simulink model "slexFMCWExample"  (R2018b)
settings: Solver=FixedStepDiscrete  StartTime=0.0  StopTime=20*64*paramFMCW.T  RelTol=1e-3  EnableMultiTasking=on
PreLoadFcn:
  | helperslexFMCWParam
undefined symbols (not defined in the file or in its folder): paramFMCW, physconst
libraries: phasedenvlib x6, phasedtxrxlib x2, phaseddetectlib x2, phasedwavlib x1, phasedmisclib x1
CloseFcn:
  | clear paramFMCW
Description:
  | FMCW Radar Range Estimation
  | 
  | This model shows how to use a FMCW radar to estimate a target's range.
settings Model: Creator=The MathWorks, Inc.  LastModifiedBy=The MathWorks, Inc.
settings DataIOCC: LimitDataPoints=on  SaveFormat=Array
settings OptimizationCC: LifeSpan=inf
settings DebuggingCC: ReadBeforeWriteMsg=DisableAll  WriteAfterWriteMsg=DisableAll  WriteAfterReadMsg=DisableAll  UnderspecifiedInitializationDetection=Classic  MergeDetectMultiDrivingBlocksExec=none  SolverPrmCheckMsg=warning  MultiTaskDSMMsg=none  AllowSymbolicDim=off  SFUnexpectedBacktrackingDiag=warning  SFNoUnconditionalDefaultTransitionDiag=warning  SFExecutionAtInitializationDiag=none
settings HardwareCC: ProdBitPerPointer=32  ProdBitPerSizeT=32  ProdBitPerPtrDiffT=32  ProdLargestAtomicFloat=None  ProdIntDivRoundTo=Undefined  ProdEndianess=Unspecified  ProdWordSize=32  ProdHWDeviceType=32-bit Generic
settings ModelReferenceCC: UpdateModelReferenceTargets=IfOutOfDate  PropagateSignalLabelsOutOfModel=off
settings SFSimCC: SFSimEcho=off  SimUseLocalCustomCode=off
settings RTWCC: RTWUseLocalCustomCode=off
settings CodeAppCC: StateflowObjectComments=on
settings GRTTargetCC: TargetLangStandard=C89/C90 (ANSI)  GeneratePreprocessorConditionals=Disable all
settings ConfigComp: CovMetricSettings=dw  CovHtmlReporting=on  CovSaveCumulativeToWorkspaceVar=on  CovSaveSingleToWorkspaceVar=on  CovExternalEMLEnable=off  CovSFcnEnable=off

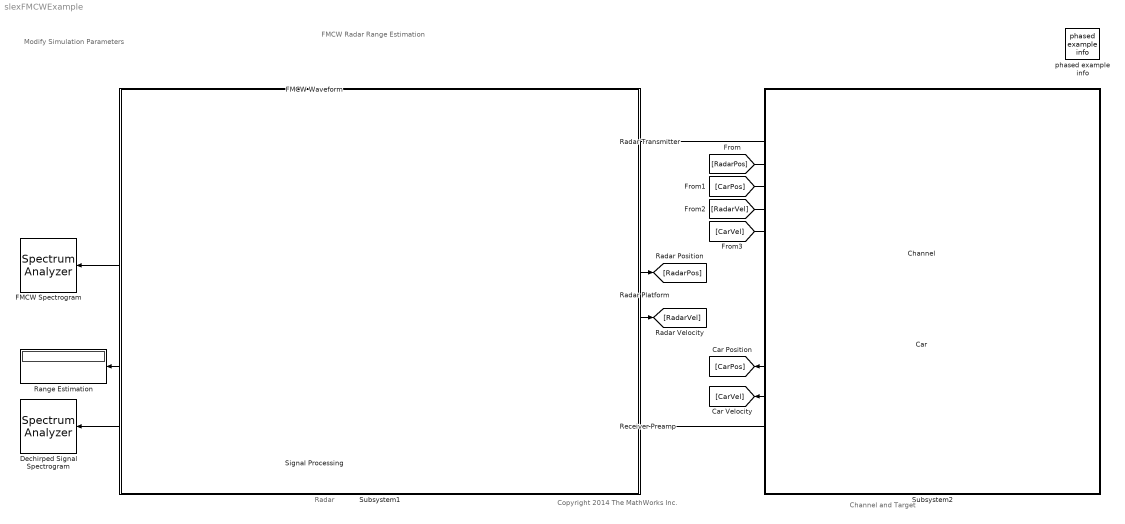
== system slexFMCWExample ==
  note: Copyright 2014 The MathWorks Inc.
  note: Radar
  note: Channel and Target
  note: FMCW Radar Range Estimation
  note: Modify Simulation Parameters
  Car : Subsystem
      mask Display:
      | disp('Car')
      | port_label('output',1,'Pos')
      | port_label('output',2,'Vel')
      | port_label('output',3,'Sig')
  Channel : Subsystem  VariantControlMode=Label  Variant=on  LabelModeActiveChoice=FreeSpace  mask{ChannelSelection=Free space}
      mask prompts: ChannelSelection "Propagation Channel"
      mask init:
      | cstr = get_param(gcb,'ChannelSelection');
      | if strcmp(cstr,'Free space')
      |     set_param(gcb,'OverrideUsingVariant','FreeSpace');
      | else
      |     set_param(gcb,'OverrideUsingVariant','TwoRay');
      | end
      mask TypeOptions ChannelSelection: Free space | Two-ray
      mask DialogControl DescGroupVar Prompt: Channel
      mask DialogControl DescTextVar Prompt: Propagation channel between the radar and the car
      mask Display:
      | port_label('output',1,'y')
      | port_label('input',1,'x')
      | port_label('input',2,'pos1')
      | port_label('input',3,'pos2')
      | port_label('input',4,'vel1')
      | port_label('input',5,'vel2')
      | disp('Channel')
  Dechirped Signal Spectrogram : SpectrumAnalyzer
  FMCW Spectrogram : SpectrumAnalyzer
  FMCW Waveform : phasedwavlib/FMCW Waveform  SampleRate=paramFMCW.Fs  SweepTime=paramFMCW.T  SweepBandwidth=paramFMCW.Fs  SweepDirection=Up  SweepInterval=Symmetric  OutputFormat=Sweeps  NumSamples=100  NumSweeps=1  SimulateUsing=Interpreted execution
      settings: SourceProductName=Phased Array System Toolbox  SourceProductBaseCode=AR
  Radar Platform : phasedenvlib/Motion Platform  MotionModel=Velocity  InitialPosition=paramFMCW.RadarPos  InitialVelocity=[ 0; 0; 0 ]  VelocitySource=Property  Velocity=paramFMCW.RadarVel  AccelerationSource=Property  Acceleration=[0;0;0]  CustomTrajectory=[ 0, 0, 0, 0, 0, 0, 0; 1, 0, 0, 0, 0, 0, 0 ]  ScanMode=None  InitialScanAngle=0  AzimuthSpan=[ -60, 60 ]  AzimuthScanRate=10  InitialOrientationAxes=eye( 3 )  OrientationAxesOutputPort=off  ElapsedTimeSource=Auto  SampleRateFromInputCheckbox=on  SampleRate=1e6  SimulateUsing=Interpreted execution
      settings: SourceProductName=Phased Array System Toolbox  SourceProductBaseCode=AR
  Radar Transmitter : phasedtxrxlib/Transmitter  PeakPower=paramFMCW.ppow  Gain=paramFMCW.TxGain  LossFactor=0  InUseOutputPort=off  CoherentOnTransmit=on  PhaseNoiseOutputPort=off  SeedSource=Auto  Seed=0  SimulateUsing=Interpreted execution
      settings: SourceProductName=Phased Array System Toolbox  SourceProductBaseCode=AR
  Range Estimation : Display
  Receiver Preamp : phasedtxrxlib/Receiver Preamp  Gain=paramFMCW.RxGain  LossFactor=0  NoiseMethod=Noise temperature  NoiseFigure=paramFMCW.NF  ReferenceTemperature=290  SampleRateFromInputCheckbox=on  SampleRate=1e6  NoisePower=0  EnableInputPort=off  PhaseNoiseInputPort=off  SeedSource=Auto  Seed=0  SimulateUsing=Interpreted execution
      settings: SourceProductName=Phased Array System Toolbox  SourceProductBaseCode=AR
  Signal Processing : Subsystem
      mask Display:
      | disp('Signal Processing')
      | port_label('input',1,'Ref')
      | port_label('input',2,'Echo')
      | port_label('output',1,'Rng')
      | port_label('output',2,'Dechirped')
  Subsystem1 : Subsystem
  Subsystem2 : Subsystem
  phased example info : phasedmisclib/phased example info  SystemSampleTime=-1
      settings: SourceProductName=Phased Array System Toolbox  SourceProductBaseCode=AR
  wires:
  FMCW Waveform/1 -> Signal Processing/1(In1), FMCW Spectrogram/1, Radar Transmitter/1
  Radar Platform/1 -> [RadarPos]
  Radar Platform/2 -> [RadarVel]
  Car/1(Out1) -> [CarPos]
  Car/2(Out2) -> [CarVel]
  Car/3(Out3) -> Receiver Preamp/1
  Receiver Preamp/1 -> Signal Processing/2(In2)
  Signal Processing/1(Out1) -> Range Estimation/1
  Signal Processing/2(Out2) -> Dechirped Signal Spectrogram/1
  Radar Transmitter/1 -> Channel/1(In1)
  [RadarPos] -> Channel/2(In2)
  [CarPos] -> Channel/3(In3)
  [RadarVel] -> Channel/4(In4)
  [CarVel] -> Channel/5(In5)
  Channel/1(Out1) -> Car/1(In1)

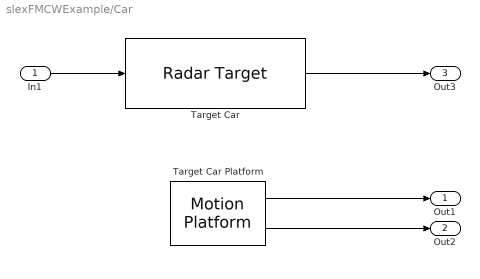
== system slexFMCWExample/Car ==
  In1 : Inport
  Target Car : phasedenvlib/Radar Target  EnablePolarization=off  Mode=Monostatic  MeanRCSSource=Property  ScatteringMatrixSource=Property  MeanRCS=paramFMCW.RCS  ScatteringMatrix=eye( 2 )  Model=Nonfluctuating  PropagationSpeed=paramFMCW.C  OperatingFrequency=paramFMCW.Fc  SeedSource=Auto  Seed=0  SimulateUsing=Interpreted execution
      settings: SourceProductName=Phased Array System Toolbox  SourceProductBaseCode=AR
  Target Car Platform : phasedenvlib/Motion Platform  MotionModel=Velocity  InitialPosition=paramFMCW.CarPos  InitialVelocity=[ 0; 0; 0 ]  VelocitySource=Property  Velocity=paramFMCW.CarVel  AccelerationSource=Property  Acceleration=[0;0;0]  CustomTrajectory=[ 0, 0, 0, 0, 0, 0, 0; 1, 0, 0, 0, 0, 0, 0 ]  ScanMode=None  InitialScanAngle=0  AzimuthSpan=[ -60, 60 ]  AzimuthScanRate=10  InitialOrientationAxes=eye( 3 )  OrientationAxesOutputPort=off  ElapsedTimeSource=Auto  SampleRateFromInputCheckbox=on  SampleRate=1e6  SimulateUsing=Interpreted execution
      settings: SourceProductName=Phased Array System Toolbox  SourceProductBaseCode=AR
  Out1 : Outport
  Out2 : Outport  Port=2
  Out3 : Outport  Port=3
  wires:
  Target Car/1 -> Out3/1
  In1/1 -> Target Car/1
  Target Car Platform/1 -> Out1/1
  Target Car Platform/2 -> Out2/1

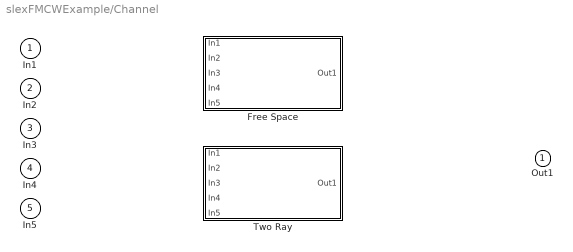
== system slexFMCWExample/Channel ==
  In1 : Inport
  In2 : Inport  Port=2
  In3 : Inport  Port=3
  In4 : Inport  Port=4
  In5 : Inport  Port=5
  Free Space : Subsystem  VariantControl=FreeSpace
      mask Display:
      | port_label('output',1,'y')
      | port_label('input',1,'x')
      | port_label('input',2,'pos1')
      | port_label('input',3,'pos2')
      | port_label('input',4,'vel1')
      | port_label('input',5,'vel2')
      | disp('Free Space')
  Two Ray : Subsystem  VariantControl=TwoRay
      mask Display:
      | port_label('output',1,'y')
      | port_label('input',1,'x')
      | port_label('input',2,'pos1')
      | port_label('input',3,'pos2')
      | port_label('input',4,'vel1')
      | port_label('input',5,'vel2')
      | disp('Two-Ray')
  Out1 : Outport

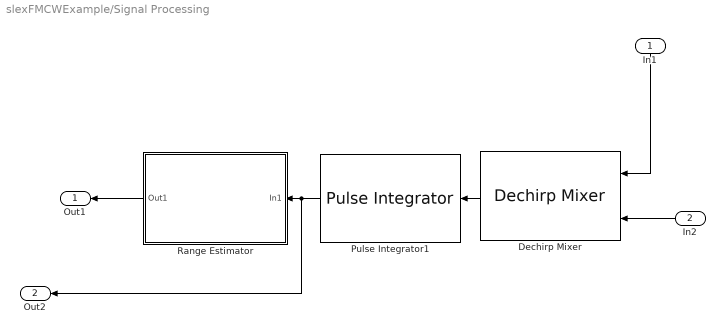
== system slexFMCWExample/Signal Processing ==
  In1 : Inport
  In2 : Inport  Port=2
  Dechirp Mixer : phaseddetectlib/Dechirp Mixer
      settings: SourceProductName=Phased Array System Toolbox  SourceProductBaseCode=AR
  Pulse Integrator1 : phaseddetectlib/Pulse Integrator  CoherentFlag=Coherent  N=64  V=0
      settings: SourceProductName=Phased Array System Toolbox  SourceProductBaseCode=AR
  Range Estimator : Subsystem  mask(Range Estimator){c=paramFMCW.C, k=paramFMCW.Fs/paramFMCW.T, N=2048}
      mask prompts: c "Propagation Speed (m/s)"; k "FMCW Sweep Slope (Hz/s)"; N "Number of FFT Points"
      mask help: Compute periodogram of the incoming signal, find the beat frequency, and convert the beat frequency to the range estimate.
      mask Display:
      | disp('Range\nEstimator')
      | port_label('input',1,'X')
      | port_label('output',1,'Rng')
  Out1 : Outport
  Out2 : Outport  Port=2
  wires:
  In1/1 -> Dechirp Mixer/1
  Dechirp Mixer/1 -> Pulse Integrator1/1
  In2/1 -> Dechirp Mixer/2
  Pulse Integrator1/1 -> Out2/1, Range Estimator/1(In1)
  Range Estimator/1(Out1) -> Out1/1

== system slexFMCWExample/Subsystem1 ==

== system slexFMCWExample/Subsystem2 ==

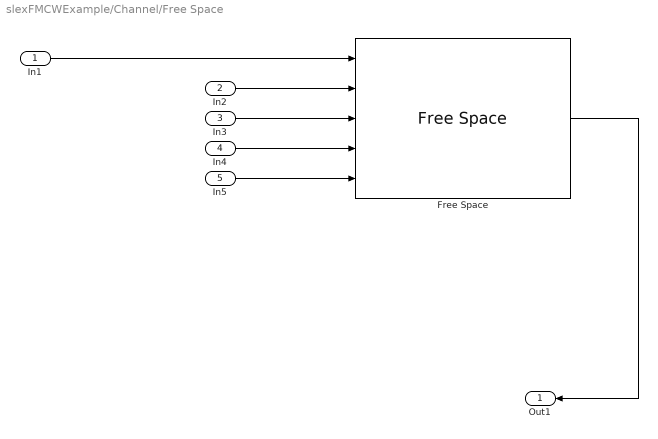
== system slexFMCWExample/Channel/Free Space ==
  In1 : Inport
  In2 : Inport  Port=2
  In3 : Inport  Port=3
  In4 : Inport  Port=4
  In5 : Inport  Port=5
  Free Space : phasedenvlib/Free Space  PropagationSpeed=paramFMCW.C  OperatingFrequency=paramFMCW.Fc  TwoWayPropagation=on  SampleRateFromInputCheckbox=on  SampleRate=1e6  MaximumDistanceSource=Property  MaximumDistance=10e3  MaximumNumInputSamplesSource=Auto  MaximumNumInputSamples=1000  SimulateUsing=Interpreted execution
      settings: SourceProductName=Phased Array System Toolbox  SourceProductBaseCode=AR
  Out1 : Outport
  wires:
  Free Space/1 -> Out1/1
  In1/1 -> Free Space/1
  In5/1 -> Free Space/5
  In4/1 -> Free Space/4
  In3/1 -> Free Space/3
  In2/1 -> Free Space/2

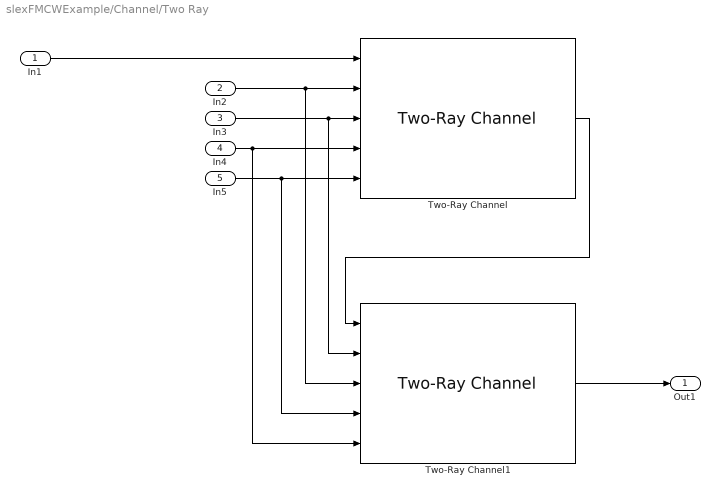
== system slexFMCWExample/Channel/Two Ray ==
  In1 : Inport
  In2 : Inport  Port=2
  In3 : Inport  Port=3
  In4 : Inport  Port=4
  In5 : Inport  Port=5
  Two-Ray Channel : phasedenvlib/Two-Ray Channel  PropagationSpeed=physconst( 'LightSpeed' )  OperatingFrequency=3e8  SpecifyAtmosphere=off  Temperature=15  DryAirPressure=101325  WaterVapourDensity=7.5  LiquidWaterDensity=0  RainRate=0  SampleRateFromInputCheckbox=on  SampleRate=1e6  GroundReflectionCoefficient=-1  GroundRelativePermittivity=15  CombinedRaysOutput=on  MaximumDistanceSource=Property  MaximumDistance=10e3  MaximumNumInputSamplesSource=Auto  MaximumNumInputSamples=1000  SimulateUsing=Interpreted execution
      settings: SourceProductName=Phased Array System Toolbox  SourceProductBaseCode=AR
  Two-Ray Channel1 : phasedenvlib/Two-Ray Channel  PropagationSpeed=physconst( 'LightSpeed' )  OperatingFrequency=3e8  SpecifyAtmosphere=off  Temperature=15  DryAirPressure=101325  WaterVapourDensity=7.5  LiquidWaterDensity=0  RainRate=0  SampleRateFromInputCheckbox=on  SampleRate=1e6  GroundReflectionCoefficient=-1  GroundRelativePermittivity=15  CombinedRaysOutput=on  MaximumDistanceSource=Property  MaximumDistance=10e3  MaximumNumInputSamplesSource=Auto  MaximumNumInputSamples=1000  SimulateUsing=Interpreted execution
      settings: SourceProductName=Phased Array System Toolbox  SourceProductBaseCode=AR
  Out1 : Outport
  wires:
  In2/1 -> Two-Ray Channel1/3, Two-Ray Channel/2
  In3/1 -> Two-Ray Channel1/2, Two-Ray Channel/3
  In4/1 -> Two-Ray Channel1/5, Two-Ray Channel/4
  In5/1 -> Two-Ray Channel1/4, Two-Ray Channel/5
  In1/1 -> Two-Ray Channel/1
  Two-Ray Channel/1 -> Two-Ray Channel1/1
  Two-Ray Channel1/1 -> Out1/1

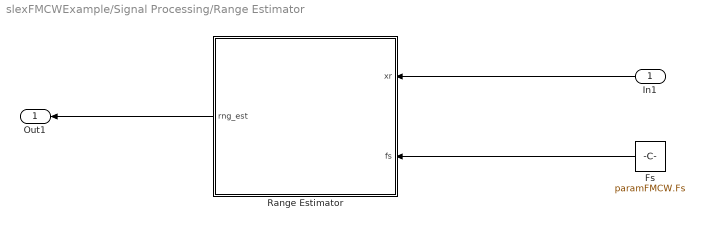
== system slexFMCWExample/Signal Processing/Range Estimator ==
  In1 : Inport
  Fs : Constant  Value=paramFMCW.Fs
  Range Estimator : MATLAB Function  TreatAsAtomicUnit=on
  Out1 : Outport
  wires:
  Range Estimator/1(rng_est) -> Out1/1
  In1/1 -> Range Estimator/1(xr)
  Fs/1 -> Range Estimator/2(fs)

== matlab function slexFMCWExample/Signal Processing/Range Estimator/Range Estimator ==
  data: xr input; rng_est output; fs input; k parameter; c parameter; N parameter
function rng_est = fcn(xr,fs,k,c,N)
%#codegen

f = fs*(-0.5+(0:N-1)/N);
P = abs(fftshift(fft(xr,N))).^2;
[~,idx] = findpeaks(P,'NPeaks',1,'SortStr','descend');
if ~isempty(idx)
    idx2 = idx(1);
    fb_rng = f(idx2);
    rng_est = double(beat2range(fb_rng,k,c));
else
    rng_est = 0;
end
